simulink subsystem "body_mdl"  (R2023a)
settings: Solver=VariableStepAuto  StartTime=0.0  StopTime=10.0  RelTol=1e-3
model mask{obj=obj}
  mask prompts: obj "Spring Object:"
settings Model: Creator=grouleau  LastModifiedBy=grouleau

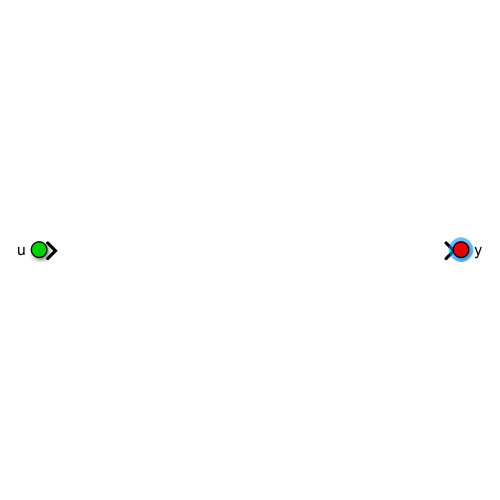
[thumbnail: Simulink's stored preview of the top-level diagram]
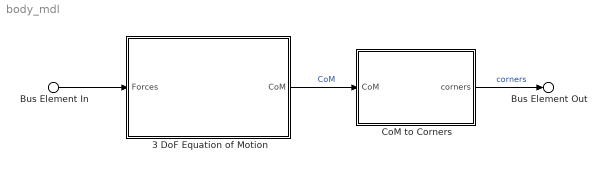
== system body_mdl ==
  Bus Element In : Inport  PortName=u
  3 DoF Equation of Motion : Subsystem
  CoM to Corners : Subsystem
  Bus Element Out : Outport  PortName=y
  wires:
  3 DoF Equation of Motion/1(CoM) -> CoM to Corners/1(CoM)  "CoM"
  Bus Element In/1 -> 3 DoF Equation of Motion/1(Forces)
  CoM to Corners/1(corners) -> Bus Element Out/1  "corners"

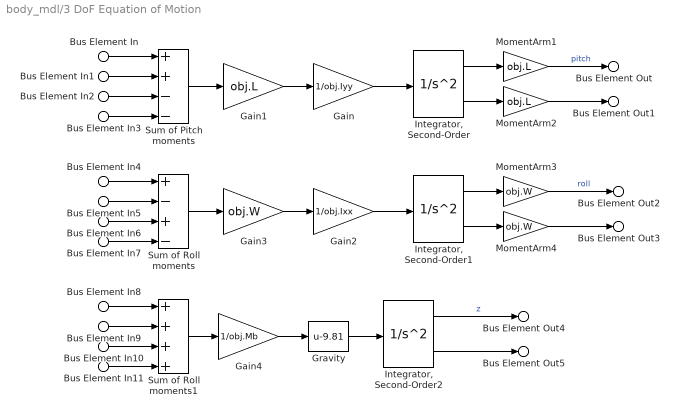
== system body_mdl/3 DoF Equation of Motion ==
  Bus Element In : Inport  PortName=Forces  Element=Forces.FrontLeft
  Bus Element In4 : Inport  PortName=Forces  Element=Forces.FrontLeft
  Bus Element In8 : Inport  PortName=Forces  Element=Forces.FrontLeft
  Bus Element In1 : Inport  PortName=Forces  Element=Forces.FrontRight
  Bus Element In5 : Inport  PortName=Forces  Element=Forces.FrontRight
  Bus Element In9 : Inport  PortName=Forces  Element=Forces.FrontRight
  Bus Element In2 : Inport  PortName=Forces  Element=Forces.RearLeft
  Bus Element In6 : Inport  PortName=Forces  Element=Forces.RearLeft
  Bus Element In10 : Inport  PortName=Forces  Element=Forces.RearLeft
  Bus Element In3 : Inport  PortName=Forces  Element=Forces.RearRight
  Bus Element In7 : Inport  PortName=Forces  Element=Forces.RearRight
  Bus Element In11 : Inport  PortName=Forces  Element=Forces.RearRight
  Gain : Gain  Gain=1/obj.Iyy
  Gain1 : Gain  Gain=obj.L
  Gain2 : Gain  Gain=1/obj.Ixx
  Gain3 : Gain  Gain=obj.W
  Gain4 : Gain  Gain=1/obj.Mb
  Gravity : Bias  Bias=-9.81  SaturateOnIntegerOverflow=off
  "Integrator, Second-Order" : SecondOrderIntegrator
  "Integrator, Second-Order1" : SecondOrderIntegrator
  "Integrator, Second-Order2" : SecondOrderIntegrator
  MomentArm1 : Gain  Gain=obj.L  SaturateOnIntegerOverflow=on  OutDataTypeStr=Inherit: Same as input  ParamDataTypeStr=Inherit: Same as input
  MomentArm2 : Gain  Gain=obj.L  SaturateOnIntegerOverflow=on  OutDataTypeStr=Inherit: Same as input  ParamDataTypeStr=Inherit: Same as input
  MomentArm3 : Gain  Gain=obj.W  SaturateOnIntegerOverflow=on  OutDataTypeStr=Inherit: Same as input  ParamDataTypeStr=Inherit: Same as input
  MomentArm4 : Gain  Gain=obj.W  SaturateOnIntegerOverflow=on  OutDataTypeStr=Inherit: Same as input  ParamDataTypeStr=Inherit: Same as input
  Sum of Pitch moments : Sum  Inputs=++--
  Sum of Roll moments : Sum  Inputs=+-+-
  Sum of Roll moments1 : Sum  Inputs=++++
  Bus Element Out : Outport  PortName=CoM  Element=pitch
  Bus Element Out1 : Outport  PortName=CoM  Element=pitchRate
  Bus Element Out2 : Outport  PortName=CoM  Element=roll
  Bus Element Out3 : Outport  PortName=CoM  Element=rollRate
  Bus Element Out4 : Outport  PortName=CoM  Element=z
  Bus Element Out5 : Outport  PortName=CoM  Element=zDot
  wires:
  "Integrator, Second-Order"/2 -> MomentArm2/1
  Bus Element In3/1 -> Sum of Pitch moments/4
  Gain1/1 -> Gain/1
  Sum of Roll moments1/1 -> Gain4/1
  "Integrator, Second-Order1"/1 -> MomentArm3/1
  Bus Element In/1 -> Sum of Pitch moments/1
  "Integrator, Second-Order1"/2 -> MomentArm4/1
  Bus Element In1/1 -> Sum of Pitch moments/2
  Bus Element In2/1 -> Sum of Pitch moments/3
  Bus Element In7/1 -> Sum of Roll moments/4
  Bus Element In6/1 -> Sum of Roll moments/3
  Gain2/1 -> "Integrator, Second-Order1"/1
  Bus Element In5/1 -> Sum of Roll moments/2
  Gain3/1 -> Gain2/1
  Sum of Roll moments/1 -> Gain3/1
  Sum of Pitch moments/1 -> Gain1/1
  Gain4/1 -> Gravity/1
  Bus Element In10/1 -> Sum of Roll moments1/3
  Bus Element In9/1 -> Sum of Roll moments1/2
  Gain/1 -> "Integrator, Second-Order"/1
  "Integrator, Second-Order"/1 -> MomentArm1/1
  "Integrator, Second-Order2"/2 -> Bus Element Out5/1
  Bus Element In11/1 -> Sum of Roll moments1/4
  "Integrator, Second-Order2"/1 -> Bus Element Out4/1  "z"
  Bus Element In4/1 -> Sum of Roll moments/1
  Bus Element In8/1 -> Sum of Roll moments1/1
  MomentArm1/1 -> Bus Element Out/1  "pitch"
  MomentArm2/1 -> Bus Element Out1/1
  MomentArm3/1 -> Bus Element Out2/1  "roll"
  MomentArm4/1 -> Bus Element Out3/1
  Gravity/1 -> "Integrator, Second-Order2"/1

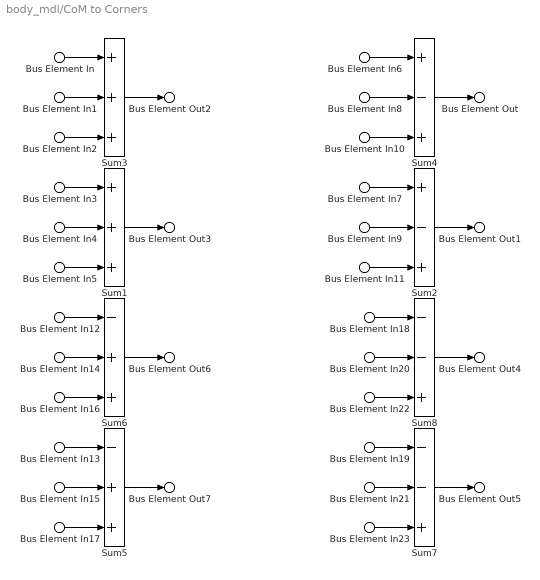
== system body_mdl/CoM to Corners ==
  Bus Element In{,6,12,18} (4 alike) : Inport  PortName=CoM  Element=pitch
  Bus Element In{1,8,14,20} (4 alike) : Inport  PortName=CoM  Element=roll
  Bus Element In{2,10,16,22} (4 alike) : Inport  PortName=CoM  Element=z
  Bus Element In{3,7,13,19} (4 alike) : Inport  PortName=CoM  Element=pitchRate
  Bus Element In{4,9,15,21} (4 alike) : Inport  PortName=CoM  Element=rollRate
  Bus Element In{5,11,17,23} (4 alike) : Inport  PortName=CoM  Element=zDot
  Sum1 : Sum  Inputs=+++  InputSameDT=on  SaturateOnIntegerOverflow=on  OutDataTypeStr=Inherit: Same as first input
  Sum2 : Sum  Inputs=+-+  InputSameDT=on  SaturateOnIntegerOverflow=on  OutDataTypeStr=Inherit: Same as first input
  Sum3 : Sum  Inputs=+++  InputSameDT=on  SaturateOnIntegerOverflow=on  OutDataTypeStr=Inherit: Same as first input
  Sum4 : Sum  Inputs=+-+  InputSameDT=on  SaturateOnIntegerOverflow=on  OutDataTypeStr=Inherit: Same as first input
  Sum5 : Sum  Inputs=-++  InputSameDT=on  SaturateOnIntegerOverflow=on  OutDataTypeStr=Inherit: Same as first input
  Sum6 : Sum  Inputs=-++  InputSameDT=on  SaturateOnIntegerOverflow=on  OutDataTypeStr=Inherit: Same as first input
  Sum7 : Sum  Inputs=--+  InputSameDT=on  SaturateOnIntegerOverflow=on  OutDataTypeStr=Inherit: Same as first input
  Sum8 : Sum  Inputs=--+  InputSameDT=on  SaturateOnIntegerOverflow=on  OutDataTypeStr=Inherit: Same as first input
  Bus Element Out2 : Outport  PortName=corners  Element=FrontLeft.z
  Bus Element Out3 : Outport  PortName=corners  Element=FrontLeft.zDot
  Bus Element Out6 : Outport  PortName=corners  Element=RearLeft.z
  Bus Element Out7 : Outport  PortName=corners  Element=RearLeft.zDot
  Bus Element Out : Outport  PortName=corners  Element=FrontRight.z
  Bus Element Out1 : Outport  PortName=corners  Element=FrontRight.zDot
  Bus Element Out4 : Outport  PortName=corners  Element=RearRight.z
  Bus Element Out5 : Outport  PortName=corners  Element=RearRight.zDot
  wires:
  Bus Element In/1 -> Sum3/1
  Bus Element In1/1 -> Sum3/2
  Bus Element In2/1 -> Sum3/3
  Sum3/1 -> Bus Element Out2/1
  Bus Element In5/1 -> Sum1/3
  Bus Element In4/1 -> Sum1/2
  Bus Element In3/1 -> Sum1/1
  Sum1/1 -> Bus Element Out3/1
  Bus Element In7/1 -> Sum2/1
  Bus Element In9/1 -> Sum2/2
  Bus Element In11/1 -> Sum2/3
  Bus Element In10/1 -> Sum4/3
  Bus Element In8/1 -> Sum4/2
  Bus Element In6/1 -> Sum4/1
  Sum4/1 -> Bus Element Out/1
  Sum2/1 -> Bus Element Out1/1
  Bus Element In13/1 -> Sum5/1
  Bus Element In15/1 -> Sum5/2
  Bus Element In17/1 -> Sum5/3
  Bus Element In16/1 -> Sum6/3
  Bus Element In14/1 -> Sum6/2
  Bus Element In12/1 -> Sum6/1
  Sum6/1 -> Bus Element Out6/1
  Sum5/1 -> Bus Element Out7/1
  Bus Element In18/1 -> Sum8/1
  Bus Element In20/1 -> Sum8/2
  Bus Element In22/1 -> Sum8/3
  Bus Element In23/1 -> Sum7/3
  Bus Element In21/1 -> Sum7/2
  Bus Element In19/1 -> Sum7/1
  Sum8/1 -> Bus Element Out4/1
  Sum7/1 -> Bus Element Out5/1
